simulink model "inverter_three_phase"  (R2015a)
settings: Solver=ode45  StartTime=0.0  StopTime=0.06  MaxStep=1/1000000  RelTol=1e-3
libraries: powerlib x14, simulink x1
settings Model: Creator=Windows 10  LastModifiedBy=Windows 10

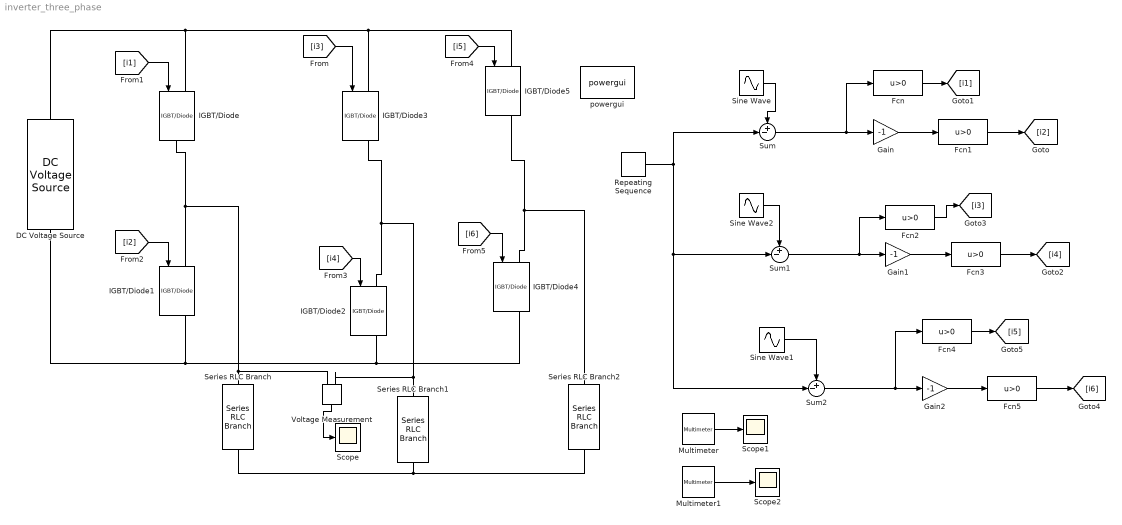
== system inverter_three_phase ==
  DC Voltage Source : powerlib/Electrical Sources/DC Voltage Source  Amplitude=565  Measurements=None
  Fcn{,1..5} (6 alike) : Fcn  Expr=u>0
  Gain : Gain  Gain=-1
  Gain1 : Gain  Gain=-1
  Gain2 : Gain  Gain=-1
  IGBT/Diode : powerlib/Power Electronics/IGBT//Diode  Ron=1e-3  Rs=1e5  Cs=inf  Measurements=off
  IGBT/Diode{1..5} (5 alike) : powerlib/Power Electronics/IGBT//Diode  Ron=1e-3  Rs=1e5  Cs=inf  Measurements=on
  Multimeter : powerlib/Measurements/Multimeter  PhasorSimulation=off  OutputType=Complex  sel=[4 5 6]  L=6  Gain=[1 1 1]  yselected={'Ib: Series RLC Branch','Ib: Series RLC Branch1','Ib: Series RLC Branch2'};  PSBOutputType=1  PSBequivalent=0  AxesSetting=[0,0.1,-100,100]  Display=0  SavedBlockNames=-11
  Multimeter1 : powerlib/Measurements/Multimeter  PhasorSimulation=off  OutputType=Complex  sel=1  L=6  Gain=1  yselected={'Ub: Series RLC Branch'};  PSBOutputType=1  PSBequivalent=0  AxesSetting=[0,0.1,-100,100]  Display=0  SavedBlockNames=-11
  Repeating Sequence : simulink/Sources/Repeating Sequence  rep_seq_t=[0 0.5 1]*1e-3  rep_seq_y=[-1 1 -1]
  Scope : Scope
  Scope1 : Scope
  Scope2 : Scope
      settings: SaveName=ScopeData2
  Series RLC Branch : powerlib/Elements/Series RLC Branch  LConnTagsString=__new0  RConnTagsString=__new0  BranchType=RL  Resistance=2  Inductance=10e-3  SetiL0=off  InitialCurrent=0  Capacitance=1e-6  Setx0=off  InitialVoltage=0  Measurements=Branch voltage and current
  Series RLC Branch1 : powerlib/Elements/Series RLC Branch  LConnTagsString=__new0  RConnTagsString=__new0  BranchType=RL  Resistance=2  Inductance=10e-3  SetiL0=off  InitialCurrent=0  Capacitance=1e-6  Setx0=off  InitialVoltage=0  Measurements=Branch voltage and current
  Series RLC Branch2 : powerlib/Elements/Series RLC Branch  LConnTagsString=__new0  RConnTagsString=__new0  BranchType=RL  Resistance=2  Inductance=10e-3  SetiL0=off  InitialCurrent=0  Capacitance=1e-6  Setx0=off  InitialVoltage=0  Measurements=Branch voltage and current
  Sine Wave : Sin  Amplitude=0.75  Frequency=2*pi*50  SampleTime=0
  Sine Wave1 : Sin  Amplitude=0.75  Frequency=2*pi*50  Phase=2*pi/3  SampleTime=0
  Sine Wave2 : Sin  Amplitude=0.75  Frequency=2*pi*50  Phase=-2*pi/3  SampleTime=0
  Sum : Sum  Inputs=+-|
  Sum1 : Sum  Inputs=+-|
  Sum2 : Sum  Inputs=+-|
  Voltage Measurement : powerlib/Measurements/Voltage Measurement  PhasorSimulation=off  OutputType=Complex  PSBequivalent=0
  powergui : powerlib/powergui  Priority=1  SimulationMode=Continuous  SolverType=Tustin/Backward Euler (TBE)  SampleTime=50e-6  frequency=60  SPID=off  DisableSnubberDevices=off  DisableRonSwitches=off  DisableVfSwitches=off  SwTol=0  DisplayEquations=off  Interpol=off  methode=off  Ts=100  FunctionMessages=off  echomessages=off  HookPort=off  EnableUseOfTLC=off  x0status=blocks  frequencyindice=0  Pbase=100e6  ErrMax=1e-4  Iterations=50  UnitsV=kV  UnitsW=MW  buscounter=0  RestoreLinks=warning  ResistiveCurrentMeasurement=off  Frange=[0:2:500]  Ylog=off  Xlog=on  ShowGrid=off  save=off  variable=ZData  structure=0  ZoomFFT=off  StartTime=0.0  cycles=1  DisplayStyle=1  fundamental=60  FreqAxis=off  MaxFrequency=1000  frequencyindicesteady=1  RmsSteady=1  display=off
  wires:
  Voltage Measurement/1 -> Scope/1
  Gain/1 -> Fcn1/1
  Fcn/1 -> [i1]
  Fcn1/1 -> [i2]
  [i1] -> IGBT/Diode/1
  [i4] -> IGBT/Diode2/1
  [i3] -> IGBT/Diode3/1
  [i2] -> IGBT/Diode1/1
  Sine Wave/1 -> Sum/1
  Sum/1 -> Fcn/1, Gain/1
  [i6] -> IGBT/Diode4/1
  [i5] -> IGBT/Diode5/1
  Gain1/1 -> Fcn3/1
  Fcn2/1 -> [i3]
  Fcn3/1 -> [i4]
  Sum1/1 -> Fcn2/1, Gain1/1
  Gain2/1 -> Fcn5/1
  Fcn4/1 -> [i5]
  Fcn5/1 -> [i6]
  Sum2/1 -> Fcn4/1, Gain2/1
  Repeating Sequence/1 -> Sum/2, Sum1/2, Sum2/2
  Multimeter/1 -> Scope1/1
  Multimeter1/1 -> Scope2/1
  Sine Wave2/1 -> Sum1/1
  Sine Wave1/1 -> Sum2/1
  connections:
  IGBT/Diode/RConn1 -- Voltage Measurement/LConn1 -- Series RLC Branch/LConn1 -- IGBT/Diode1/LConn1
  IGBT/Diode3/RConn1 -- Voltage Measurement/LConn2 -- Series RLC Branch1/LConn1 -- IGBT/Diode2/LConn1
  IGBT/Diode1/RConn1 -- DC Voltage Source/LConn1 -- IGBT/Diode4/RConn1 -- IGBT/Diode2/RConn1
  IGBT/Diode/LConn1 -- IGBT/Diode5/LConn1 -- IGBT/Diode3/LConn1 -- DC Voltage Source/RConn1
  IGBT/Diode5/RConn1 -- Series RLC Branch2/LConn1 -- IGBT/Diode4/LConn1
  Series RLC Branch/RConn1 -- Series RLC Branch1/RConn1 -- Series RLC Branch2/RConn1
